simulink subsystem "Controller"  (R2022a)
settings: Solver=VariableStepAuto  StartTime=0.0  StopTime=10.0  RelTol=1e-3
settings Model: Creator=intel  LastModifiedBy=intel

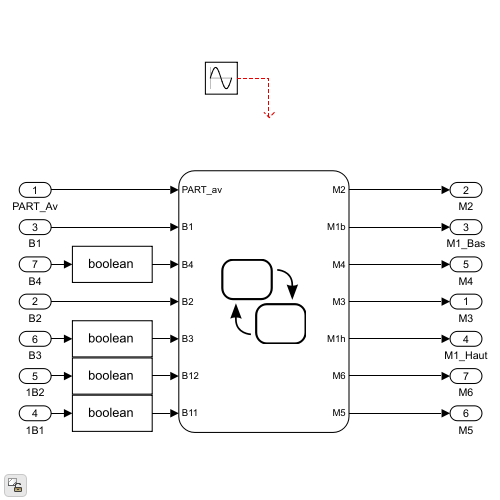
[thumbnail: Simulink's stored preview of the top-level diagram]
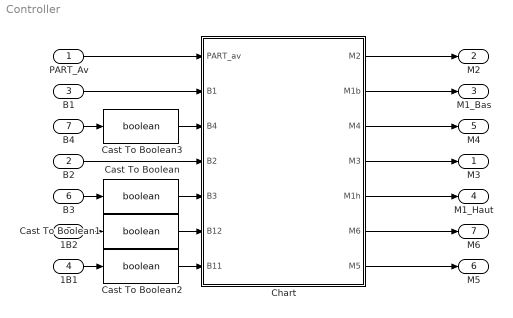
== system Controller ==
  PART_Av : Inport
  B2 : Inport  Port=2
  B1 : Inport  Port=3
  1B1 : Inport  Port=4
  1B2 : Inport  Port=5
  B3 : Inport  Port=6
  B4 : Inport  Port=7
  Cast To Boolean{,1..3} (4 alike) : DataTypeConversion  OutDataTypeStr=boolean  SaturateOnIntegerOverflow=off  RndMeth=Floor
  Chart : Stateflow chart  TreatAsAtomicUnit=on
  M3 : Outport
  M2 : Outport  Port=2
  M1_Bas : Outport  Port=3
  M1_Haut : Outport  Port=4
  M4 : Outport  Port=5
  M5 : Outport  Port=6
  M6 : Outport  Port=7
  wires:
  PART_Av/1 -> Chart/1(PART_av)
  B1/1 -> Chart/2(B1)
  B4/1 -> Cast To Boolean3/1
  B2/1 -> Chart/4(B2)
  B3/1 -> Cast To Boolean/1
  1B2/1 -> Cast To Boolean1/1
  1B1/1 -> Cast To Boolean2/1
  Chart/1(M2) -> M2/1
  Chart/2(M1b) -> M1_Bas/1
  Chart/5(M1h) -> M1_Haut/1
  Chart/3(M4) -> M4/1
  Chart/7(M5) -> M5/1
  Chart/6(M6) -> M6/1
  Chart/4(M3) -> M3/1
  Cast To Boolean/1 -> Chart/5(B3)
  Cast To Boolean1/1 -> Chart/6(B12)
  Cast To Boolean2/1 -> Chart/7(B11)
  Cast To Boolean3/1 -> Chart/3(B4)

== stateflow chart Controller/Chart ==
  state X1
  state Xf
    SS1=false;
    SS2=false;
    SS3=false;
  state X2
    entry: M2=true;
  state X3
    entry: M2=false;
  state S
    state S3 [parallel]
      settings: executionOrder=1
      state X9
      state X10
        entry: M3=true;
        entry: M4=true;
        entry: M1b=true;
      state X11
        entry: M3=true;
        entry: M4=true;
        entry: M1b=false;
        entry: M1h=true;
      state X12
        SS3=true;
        entry:M4=false;
        entry: M3=false;
        entry: M1h=false;
      (default) -> X9
      X9 -> X10 [order 1] : [B2]
      X9 -> X12 [order 2] : [~B2]
      X10 -> X11 : [B12]
      X11 -> X12 : [B11]
    state S1 [parallel]
      settings: executionOrder=3
      state X4
        entry: M6=true;
      state X5
        SS1=true;
        entry: M6=false;
      (default) -> X4
      X4 -> X5 : after(5,sec)
    state S2 [parallel]
      settings: executionOrder=2
      state X6
      state X7
        entry: M5=1;
      state X8
        SS2=true;
        entry: M5=0;
      (default) -> X6
      X6 -> X7 [order 1] : [B1]
      X6 -> X8 [order 2] : [~B1]
      X7 -> X8 : [B4]
  (default) -> X1
  Xf -> X1
  S -> Xf : [SS1&SS2&SS3]
  X1 -> X2 : [(PART_av | B1 | B2) & (~B4)]
  X2 -> X3 : [B3]
  X3 -> S : after(5,sec)
  data: PART_av input; M2 output; B1 input; B4 input; B2 input; M1b output; M4 output; M3 output; M1h output; M6 output; M5 output; SS1 local =false; SS2 local =false; SS3 local =false; B3 input; B12 input; B11 input
